simulink model "kinctrltetis"  (Simulink 8.1)
settings: Solver=ode45  StartTime=0.0  StopTime=20.0  MaxStep=0.2  RelTol=1e-5
values from neighbouring files (symbols this model uses):
  qr = [0 -pi/4 pi/2 0 ]    [mdl_tetis.m]
libraries: roblocks x5, simulink x1
settings Model: Creator=fernando  LastModifiedBy=fernando

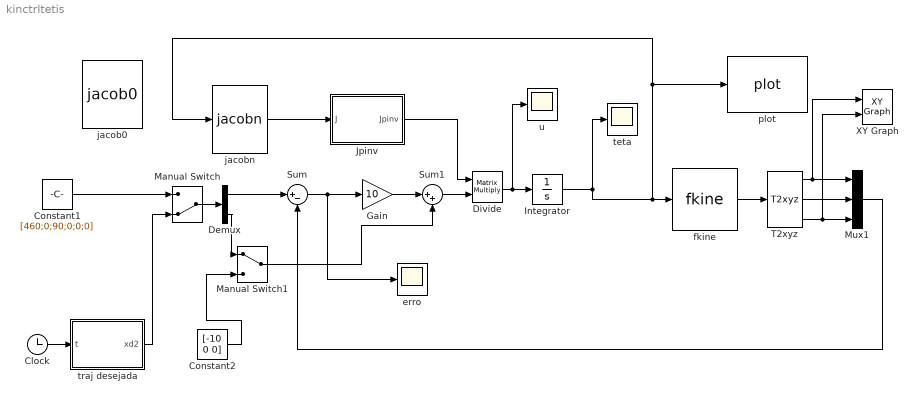
== system kinctrltetis ==
  Clock : Clock
  Constant1 : Constant  Value=[460;0;90;0;0;0]
  Constant2 : Constant  Value=[-10 0 0]
  Demux : Demux  Outputs=2
  Divide : Product  Inputs=**  Multiplication=Matrix(*)
  Gain : Gain  Gain=10
  Integrator : Integrator  InitialCondition=qr
  Jpinv : MATLAB Function  TreatAsAtomicUnit=on
  Manual Switch : ManualSwitch  CurrentSetting=0
  Manual Switch1 : ManualSwitch
  Mux1 : Mux  Inputs=3
  Sum : Sum  Inputs=|+-
  Sum1 : Sum  Inputs=|++
  T2xyz : roblocks/Transform Conversion/T2xyz
  XY Graph : simulink/Sinks/XY Graph  xmin=-0  xmax=800  ymin=-100  ymax=300  st=-1
  erro : Scope
      settings: TimeRange=20  YMin=-0.002  YMax=0.0025  SaveName=ScopeData2
  fkine : roblocks/Kinematics/fkine  robot=Tetis
  "jacob0 " : roblocks/Kinematics/jacob0   robot=robot
  jacobn : roblocks/Kinematics/jacobn  robot=Tetis
  plot : roblocks/Robot Graphics/plot  robot=Tetis  fps=20  holdplot=on
  teta : Scope
      settings: TimeRange=20  YMin=-0.8  YMax=1.6
  traj desejada : MATLAB Function  TreatAsAtomicUnit=on
  u : Scope
      settings: YMin=-0.9  YMax=0.8
  wires:
  Integrator/1 -> plot/1, jacobn/1, fkine/1, teta/1
  Divide/1 -> Integrator/1, u/1
  Jpinv/1(Jpinv) -> Divide/1
  Sum/1 -> Gain/1, erro/1
  fkine/1 -> T2xyz/1
  T2xyz/1 -> Mux1/1, XY Graph/1
  T2xyz/2 -> Mux1/2
  T2xyz/3 -> Mux1/3, XY Graph/2
  Mux1/1 -> Sum/2
  jacobn/1 -> Jpinv/1(J)
  Constant1/1 -> Manual Switch/1
  Clock/1 -> traj desejada/1(t)
  traj desejada/1(xd2) -> Manual Switch/2
  Manual Switch/1 -> Demux/1
  Demux/1 -> Sum/1
  Gain/1 -> Sum1/1
  Sum1/1 -> Divide/2
  Manual Switch1/1 -> Sum1/2
  Demux/2 -> Manual Switch1/1
  Constant2/1 -> Manual Switch1/2

== matlab function Jpinv ==
  data: J input double; Jpinv output double
function Jpinv = fcn(J)
%#codegen

Ja=[J(1:3,:)]; %;J(6,:)];
Jpinv = pinv(Ja);

== matlab function traj desejada ==
  data: t input double; xd2 output double
function xd2  = fcn(t)
%#codegen

wn=2*pi/10;

%xd= [(200) 0 (250)]';
%xddot= [0 0 0]';
%xd= [(75*sin(wn*t)+228) 0 (75*cos(wn*t)+278)]';
%xddot= [75*wn*cos(wn*t) 0 -75*wn*sin(wn*t)]';

xd= [(75*(sin(wn*t)+sin(4*wn*t))+460) 0 (75*(cos(wn*t)+cos(4*wn*t))+90)]';
xddot= [75*(wn*cos(wn*t)+4*wn*cos(4*wn*t)) 0 -75*(wn*sin(wn*t)+4*wn*sin(4*wn*t))]';

xd2=[xd;xddot];
